simulink model "pendulum"  (R2025b)
settings: Solver=VariableStepAuto  StartTime=0.0  StopTime=10  RelTol=1e-3
values from neighbouring files (symbols this model uses):
  K = place(A, B, p)    [IP2_init.m]    (also in IP3_init.m; IP4_init.m; IP_init.m; motor_init.m = 0.09)
  L = place(A', C', p)'    [IP2_init.m]    (also in motor_init.m = 0.0005; velocity_robot_rcm_ur5e_init.m = 0.3)
undefined symbols (not defined in the file or in its folder): Continuous, Kf, linsys, Time
libraries: ctrlSharedLib x1
settings Model: Creator=Junch  LastModifiedBy=Junch

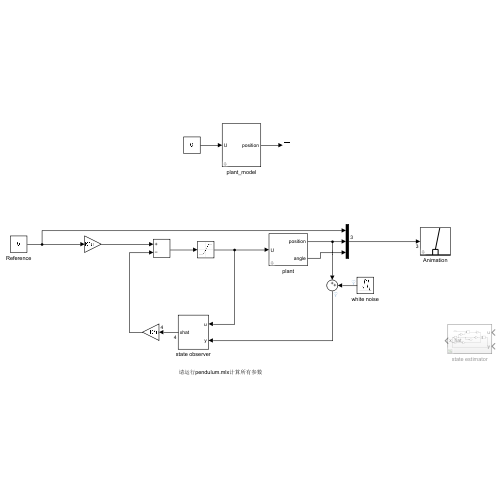
[thumbnail: Simulink's stored preview of the top-level diagram]
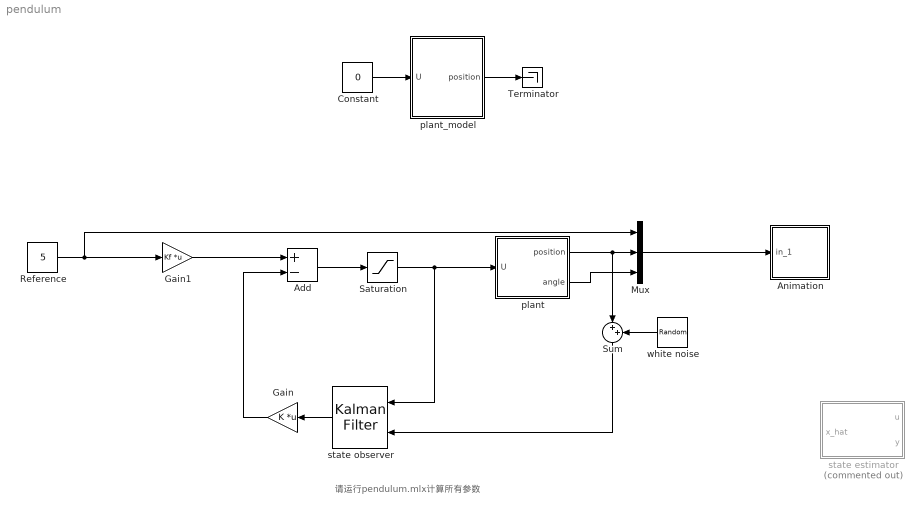
== system pendulum ==
  note: 请运行pendulum.mlx计算所有参数
  Add : Sum  Inputs=+-
  Animation : Subsystem  mask(Pendulum plot){RefBlock=Reference}
      mask prompts: RefBlock "DC reference signal block name:"
      mask help: Pendulum plot
      mask Help: Pendulum animation function using Handle graphics.
      mask Display: plot([-10 10],[0 0],[-2 -2 2 2],[0 1 1 0],[0 3],[1 5])
  Constant : Constant  Value=0
  Gain : Gain  Gain=K  Multiplication=Matrix(K*u)
  Gain1 : Gain  Gain=Kf  Multiplication=Matrix(K*u)
  Mux : Mux  Inputs=3
  Reference : Constant  Value=5
  Saturation : Saturate  UpperLimit=10  LowerLimit=-10
  Sum : Sum  Inputs=|++
  Terminator : Terminator
  plant : Subsystem  mask(Inverted Pendulum Dynamics){Mcart=0.455, m=0.21, l=0.61/2, g=9.8}
      mask prompts: Mcart "Mass of cart (kg):"; m "Mass of pendulum (kg):"; l "Distance to pendulum center of mass (m):"; g "Acceleration of gravity (m/s^2):"
      mask help: Masked subsystem containing nonlinear dynamics of inverted pendulum on a cart.
      mask Help: Nonlinear dynamics of inverted pendulum on cart.
  plant_model : Subsystem  mask(Inverted Pendulum Dynamics){Mcart=0.455, m=0.21, l=0.61/2, g=9.8}
      mask prompts: Mcart "Mass of cart (kg):"; m "Mass of pendulum (kg):"; l "Distance to pendulum center of mass (m):"; g "Acceleration of gravity (m/s^2):"
      mask help: Masked subsystem containing nonlinear dynamics of inverted pendulum on a cart.
      mask Help: Nonlinear dynamics of inverted pendulum on cart.
  state estimator : Subsystem  Commented=on
  state observer : ctrlSharedLib/Kalman Filter  TimeDomain=Continuous-Time  UseCurrentEstimator=on  ModelSource=Individual A, B, C, D matrices  ModelSourceVariable=ss(0.95,1,1,0,1)  A=linsys.A  B=linsys.B  C=linsys.C  D=linsys.D  NumberOfStates=1  NumberOfInputs=1  NumberOfOutputs=1  InitialEstimateSource=Dialog  X0=0  P0=10  UseK=off  UseGH=off  NumberOfProcessNoiseInputs=1  G=1  TimeInvariantG=on  H=0  TimeInvariantH=on  Q=0.05  TimeInvariantQ=on  R=1e-4  TimeInvariantR=on  N=0  TimeInvariantN=on  AddInputPort=on  AddEnablePort=off  OutputEstimatedY=off  OutputP=off  Ts=-1
  white noise : RandomNumber  Variance=1e-4  SampleTime=1e-3
  wires:
  Reference/1 -> Gain1/1, Mux/1
  plant/1(position) -> Sum/1, Mux/2
  Gain/1 -> Add/2
  Add/1 -> Saturation/1
  plant/2(angle) -> Mux/3
  Mux/1 -> Animation/1(in_1)
  Constant/1 -> plant_model/1(U)
  plant_model/1(position) -> Terminator/1
  Sum/1 -> state observer/2
  state observer/1 -> Gain/1
  white noise/1 -> Sum/2
  Gain1/1 -> Add/1
  Saturation/1 -> state observer/1, plant/1(U)

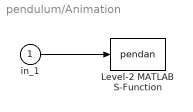
== system pendulum/Animation ==
  in_1 : Inport
  Level-2 MATLAB S-Function : M-S-Function  FunctionName=pendan  Parameters=RefBlock
  wires:
  in_1/1 -> Level-2 MATLAB S-Function/1

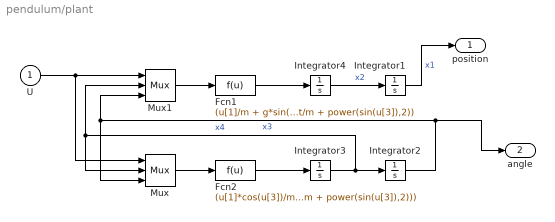
== system pendulum/plant ==
  U : Inport  Unit=N
  Fcn1 : Fcn  Expr=(u[1]/m + g*sin(u[3])*cos(u[3]) - l*power(u[2],2)*sin(u[3]))/(Mcart/m + power(sin(u[3]),2))
  Fcn2 : Fcn  Expr=(u[1]*cos(u[3])/m + (Mcart+m)*g*sin(u[3])/m - l*power(u[2],2)*sin(u[3])*cos(u[3]))/(l*(Mcart/m + power(sin(u[3]),2)))
  Integrator1 : Integrator  ContinuousStateAttributes='x'
  Integrator2 : Integrator  ContinuousStateAttributes='theta'
  Integrator3 : Integrator  ContinuousStateAttributes='omega'
  Integrator4 : Integrator  ContinuousStateAttributes='v'
  Mux : Mux  Inputs=3
  Mux1 : Mux  Inputs=3
  position : Outport
  angle : Outport  Port=2
  wires:
  Integrator1/1 -> position/1  "x1"
  Fcn2/1 -> Integrator3/1
  Mux/1 -> Fcn2/1
  Mux1/1 -> Fcn1/1
  Fcn1/1 -> Integrator4/1
  Integrator4/1 -> Integrator1/1  "x2"
  U/1 -> Mux1/1, Mux/1
  Integrator3/1 -> Mux1/2, Mux/2, Integrator2/1  "x4"
  Integrator2/1 -> angle/1, Mux1/3, Mux/3  "x3"

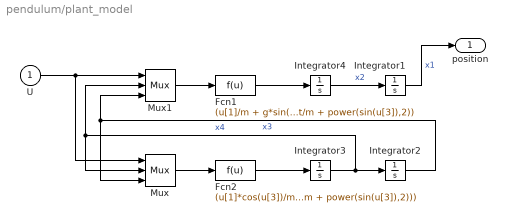
== system pendulum/plant_model ==
  U : Inport  Unit=N
  Fcn1 : Fcn  Expr=(u[1]/m + g*sin(u[3])*cos(u[3]) - l*power(u[2],2)*sin(u[3]))/(Mcart/m + power(sin(u[3]),2))
  Fcn2 : Fcn  Expr=(u[1]*cos(u[3])/m + (Mcart+m)*g*sin(u[3])/m - l*power(u[2],2)*sin(u[3])*cos(u[3]))/(l*(Mcart/m + power(sin(u[3]),2)))
  Integrator1 : Integrator  ContinuousStateAttributes='x'
  Integrator2 : Integrator  ContinuousStateAttributes='theta'
  Integrator3 : Integrator  ContinuousStateAttributes='omega'
  Integrator4 : Integrator  ContinuousStateAttributes='v'
  Mux : Mux  Inputs=3
  Mux1 : Mux  Inputs=3
  position : Outport
  wires:
  Integrator1/1 -> position/1  "x1"
  Fcn2/1 -> Integrator3/1
  Mux/1 -> Fcn2/1
  Mux1/1 -> Fcn1/1
  Fcn1/1 -> Integrator4/1
  Integrator4/1 -> Integrator1/1  "x2"
  U/1 -> Mux1/1, Mux/1
  Integrator3/1 -> Mux1/2, Mux/2, Integrator2/1  "x4"
  Integrator2/1 -> Mux1/3, Mux/3  "x3"

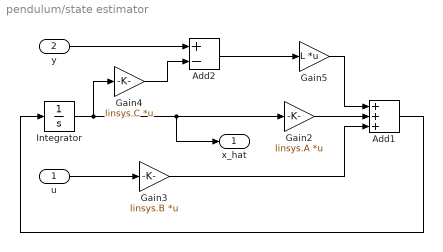
== system pendulum/state estimator ==
  u : Inport
  y : Inport  Port=2
  Add1 : Sum  Inputs=+++
  Add2 : Sum  Inputs=+-
  Gain2 : Gain  Gain=linsys.A  Multiplication=Matrix(K*u)
  Gain3 : Gain  Gain=linsys.B  Multiplication=Matrix(K*u)
  Gain4 : Gain  Gain=linsys.C  Multiplication=Matrix(K*u)
  Gain5 : Gain  Gain=L  Multiplication=Matrix(K*u)
  Integrator : Integrator
  x_hat : Outport
  wires:
  Gain3/1 -> Add1/3
  Add2/1 -> Gain5/1
  Gain2/1 -> Add1/2
  y/1 -> Add2/1
  Integrator/1 -> Gain4/1, x_hat/1, Gain2/1
  Add1/1 -> Integrator/1
  u/1 -> Gain3/1
  Gain4/1 -> Add2/2
  Gain5/1 -> Add1/1
